simulink model "pos2airgapUNITS"  (R2022b)
settings: Solver=VariableStepAuto  StartTime=0.0  StopTime=10.0  RelTol=1e-3
settings Model: Creator=USUARIO  LastModifiedBy=USUARIO

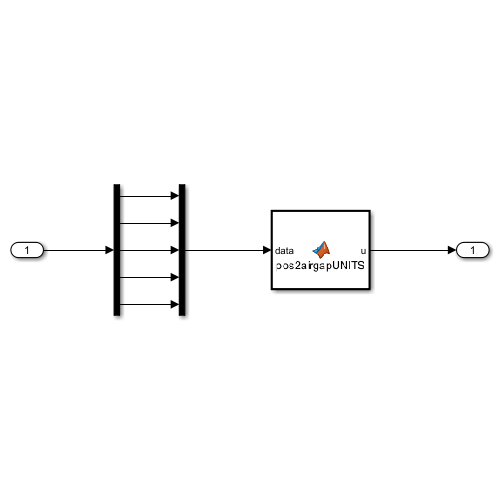
[thumbnail: Simulink's stored preview of the top-level diagram]
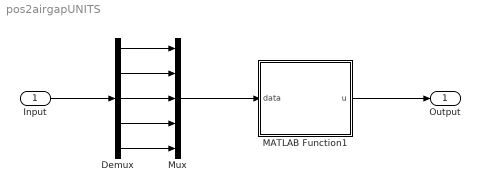
== system pos2airgapUNITS ==
  Input : Inport
  Demux : Demux  Outputs=5
  MATLAB Function1 : MATLAB Function  TreatAsAtomicUnit=on
  Mux : Mux  Inputs=5
  Output : Outport
  wires:
  Demux/1 -> Mux/1
  Demux/2 -> Mux/2
  Demux/5 -> Mux/5
  Demux/3 -> Mux/3
  Mux/1 -> MATLAB Function1/1(data)
  Demux/4 -> Mux/4
  Input/1 -> Demux/1
  MATLAB Function1/1(u) -> Output/1

== matlab function pos2airgapUNITS/MATLAB Function1 ==
  data: data input; u output
function u = pos2airgapUNITS(data)

% CONSTANTES

x_hems = [0.4475, 0.4475, 0.5465, 0.5465]; 
y_ems = [0.24253, 0.24253, 0.24253, 0.24253];
z_ems = [0.026, 0.026, 0.026, 0.026]; 

x_hems = [0.443, 0.443, 0.542, 0.542];
y_hems = [0.23686, 0.23686, 0.23686, 0.23686];
z_hems = [0.08546, 0.08546, 0.08546, 0.08546]; 

z_infr = 0.6328;

y = data(1);
z = data(2);
rotx = data(3);
roty = data(4);
rotz = data(5);



% DISTANCIAS
airgap5 = + y + y_ems(1) * cos(rotz) + x_sragy(1) * sin(rotz);
airgap6 = - y + y_ems(2) * cos(rotz) - x_sragy(2) * sin(rotz);
airgap7 = + y + y_ems(3) * cos(rotz) - x_sragy(3) * sin(rotz);
airgap8 = - y + y_ems(4) * cos(rotz) + x_sragy(4) * sin(rotz);


airgap1 =  +z - z_infr  + z_hems(1) * cos(roty) + x_hems(1) * sin(roty) - y_hems(1) * sin(rotx);
airgap2 =  +z - z_infr  + z_hems(2) * cos(roty) + x_hems(2) * sin(roty) + y_hems(2) * sin(rotx);
airgap3 =  +z - z_infr  + z_hems(3) * cos(roty) - x_hems(3) * sin(roty) - y_hems(3) * sin(rotx);
airgap4 =  +z - z_infr  + z_hems(4) * cos(roty) - x_hems(4) * sin(roty) + y_hems(4) * sin(rotx);


u =[airgap1, airgap2, airgap3, airgap4, airgap5, airgap6, airgap7, airgap8]';
